simulink model "C_PTES_sim_v2"  (R2025a)
settings: Solver=ode23tb  StartTime=0.0  StopTime=600
PreLoadFcn:
  | Load_Maps
InitFcn:
  | A_init_compressor
StopFcn:
  | % AB_plotHX
  | % AB_plotmap
model workspace (MAT data in the model file):
  Step_time = 1000
  step_time = 200
values from neighbouring files (symbols this model uses):
  DeltaW = 0    [A_init_compressor.m]    (also in B_init_compressor.m = input('Power change: '))
  Ki_tau = 23.1297    [A_init_compressor.m]    (also in B_init_compressor.m = 0.1)
  Kp_tau = 289.6844    [A_init_compressor.m]    (also in B_init_compressor.m = 1)
  omega_step = 376    [A_init_compressor.m]
  stepping_time = 100000    [A_init_compressor.m]    (also in B_init_compressor.m = input('Step time:'))
  tchange = 100000    [A_init_compressor.m]
undefined symbols (not defined in the file or in its folder): z_Qlty_CO2
libraries: simulink_extras x17, slpidlib x9
(part 1 of 3)
settings Model: Creator=mmercang  LastModifiedBy=alpalbay
settings SolverCC: ConsecutiveZCsStepRelTol=auto  ZeroCrossAlgorithm=Adaptive  MinimalZcImpactIntegration=on
settings DataIOCC: FinalStateName=xfinal  InitialState=steady_state  LoadInitialState=on  SaveFinalState=on  SaveFormat=StructureWithTime  SaveState=on  Refine=2
settings DebuggingCC: ReadBeforeWriteMsg=DisableAll  WriteAfterWriteMsg=DisableAll  WriteAfterReadMsg=DisableAll  AlgebraicLoopMsg=none  IgnoredZcDiagnostic=none  MultiTaskDSMMsg=none
settings ModelReferenceCC: UpdateModelReferenceTargets=IfOutOfDate
settings SFSimCC: SFSimEcho=off
settings RTWCC: GPUComputeCapability=3.5
settings SimscapeCC: SimscapeLogDecimation=1  SimscapeLogDataHistory=5000

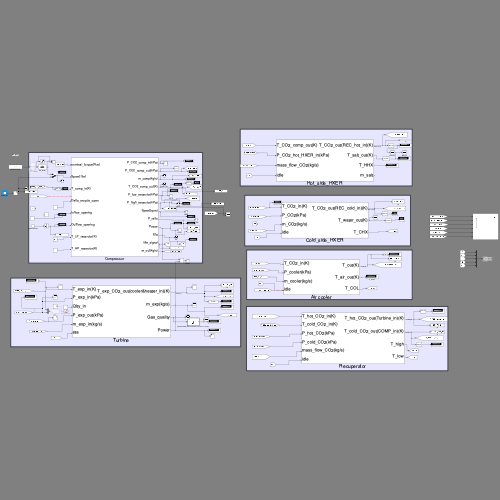
[thumbnail: Simulink's stored preview of the top-level diagram]
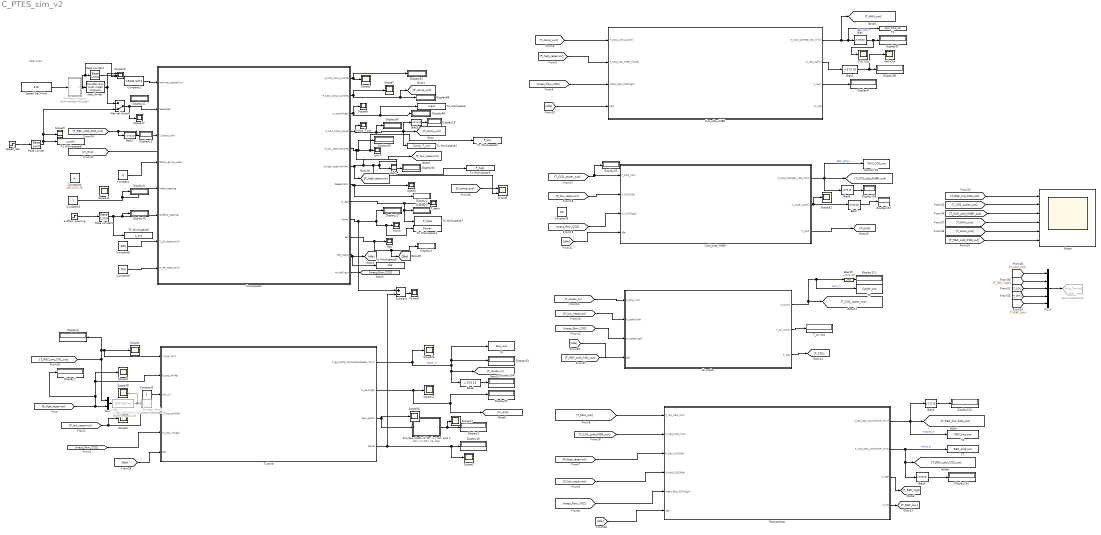
== system C_PTES_sim_v2 ==
  note: 368.2243
  Air cooler : Subsystem
  Bias{,1..8,15} (10 alike) : Bias  Bias=-273.15  SaturateOnIntegerOverflow=off
  CO2 Out : Scope
      settings: ActiveDisplayYMinimum=419.41887849810757  ActiveDisplayYMaximum=425.62012461132127  DataLoggingVariableName=ScopeData57
  Cold_side_HXER : Subsystem
  Comp T out : Scope
      settings: ActiveDisplayYMinimum=932.8388554275466  ActiveDisplayYMaximum=966.06264783948268  DataLoggingVariableName=ScopeData42
  Compressor : Subsystem
  Constant : Constant  Value=0
  Constant1 : Constant  Value=19102.6473
  Constant2 : Constant
  Constant3 : Constant
  Constant4 : Constant  Value=420+273.15
  Constant5 : Constant  Value=50
  Constant8 : Constant  Value=690
  Constant9 : Constant  Value=700
  Display{1..4,6..13,16,19..20,87..94,97..98,101..102,104,107..108,113} (31 alike) : Display
      Display12 settings: Format=bank
  Dryness check : MATLAB Function  Commented=on  TreatAsAtomicUnit=on
  "Dryness check (0 for \"x<=0\" and 1 for \"x>=1\" i.e. dry)" : MATLAB Function  TreatAsAtomicUnit=on
  Eta : Scope
      settings: ActiveDisplayYMinimum=0.8  ActiveDisplayYMaximum=1  DataLoggingVariableName=ScopeData44
  Goto17 : Goto  Commented=on  GotoTag=Avg_Temps
  High P : Scope
      settings: ActiveDisplayYMinimum=19499.01131682  ActiveDisplayYMaximum=19499.01131709  DataLoggingVariableName=ScopeData45
  Hot_side_HXER : Subsystem
  Low P : Scope
      settings: ActiveDisplayYMinimum=1661.4124691306079  ActiveDisplayYMaximum=8047.2877774228209  DataLoggingVariableName=ScopeData46
  Manual Switch : ManualSwitch  CurrentSetting=0
  Mux : Mux  Inputs=2
  Mux1 : Mux  Inputs=5
  P_ratio : Scope
      settings: ActiveDisplayYMinimum=2.5704663897454543  ActiveDisplayYMaximum=2.6288728670169967  DataLoggingVariableName=ScopeData47
  Power : Scope
      settings: ActiveDisplayYMinimum=9622.94144984568  ActiveDisplayYMaximum=9622.9443761527218  DataLoggingVariableName=ScopeData48
  Power1 : Scope
      settings: ActiveDisplayYMinimum=-764.83256469030607  ActiveDisplayYMaximum=6887.6317450574907  DataLoggingVariableName=ScopeData84
  Qlty : MATLABFcn  Commented=on  MATLABFcn=z_Qlty_CO2(u(1),u(2))
  Rate Limiter : RateLimiter
  Rate Limiter1 : RateLimiter  RisingSlewLimit=4  FallingSlewLimit=-4  InitialCondition=376  LinearizeAsGain=off
  Rate Limiter2 : RateLimiter  FallingSlewLimit=-0.01
  Recuperator : Subsystem
  Salt Out : Scope
      settings: ActiveDisplayYMinimum=549.32679199371159  ActiveDisplayYMaximum=549.32679200120469  DataLoggingVariableName=ScopeData58
  Scope : Scope  NumInputPorts=6
      settings: ActiveDisplayYMinimum=408.50778721774293  ActiveDisplayYMaximum=410.82110455322322
  Scope{1..5,7..9,11,17,22..23,26..28,51} (16 alike) : Scope
      Scope1 settings: ActiveDisplayYMinimum=354.53484488928774  ActiveDisplayYMaximum=416.54773222280147
      Scope11 settings: ActiveDisplayYMinimum=0.043750000000000011  ActiveDisplayYMaximum=1.10625  DataLoggingVariableName=ScopeData15
      Scope17 settings: ActiveDisplayYMinimum=346.2691444179722  ActiveDisplayYMaximum=643.57770023825037  DataLoggingVariableName=ScopeData49
      Scope2 settings: ActiveDisplayYMinimum=3609.0647035085312  ActiveDisplayYMaximum=3633.4611371786241
      Scope22 settings: ActiveDisplayYMinimum=53.375645074893505  ActiveDisplayYMaximum=53.375742212262359  DataLoggingVariableName=ScopeData5
      Scope23 settings: ActiveDisplayYMinimum=249.61773578013822  ActiveDisplayYMaximum=330.2583181291364  DataLoggingVariableName=ScopeData6
      Scope26 settings: ActiveDisplayYMinimum=-1  ActiveDisplayYMaximum=1
      Scope27 settings: ActiveDisplayYMinimum=-1  ActiveDisplayYMaximum=1  DataLoggingVariableName=ScopeData2
      Scope28 settings: ActiveDisplayYMinimum=-1  ActiveDisplayYMaximum=1  DataLoggingVariableName=ScopeData3
      Scope3 settings: ActiveDisplayYMinimum=6922.0923934778948  ActiveDisplayYMaximum=12119.561569977996  DataLoggingVariableName=ScopeData50
      Scope4 settings: ActiveDisplayYMinimum=19499.011316899083  ActiveDisplayYMaximum=19499.011316899174  DataLoggingVariableName=ScopeData5
      Scope5 settings: ActiveDisplayYMinimum=7403.99999999722  ActiveDisplayYMaximum=7404.0000000235223  DataLoggingVariableName=ScopeData6
      Scope51 settings: ActiveDisplayYMinimum=252.25553854956786  ActiveDisplayYMaximum=331.783751710615  DataLoggingVariableName=ScopeData2
      Scope7 settings: ActiveDisplayYMinimum=-9616.8305551512967  ActiveDisplayYMaximum=198282.22438144876  DataLoggingVariableName=ScopeData52
      Scope8 settings: ActiveDisplayYMinimum=53.375694282294106  ActiveDisplayYMaximum=53.37575539188817  DataLoggingVariableName=ScopeData53
      Scope9 settings: ActiveDisplayYMinimum=276  ActiveDisplayYMaximum=476  DataLoggingVariableName=ScopeData85
  Scope10 : Scope  NumInputPorts=3
      settings: ActiveDisplayYMinimum=375.99999999999989  ActiveDisplayYMaximum=376.00000000000011  DataLoggingVariableName=ScopeData10
  Scope6 : Scope  NumInputPorts=2
      settings: ActiveDisplayYMinimum=724.91071659726686  ActiveDisplayYMaximum=20997.430200370087  DataLoggingVariableName=ScopeData55
  Shutdown Signal : Subsystem  Commented=through
  Speed : Scope
      settings: ActiveDisplayYMinimum=375.99998147375209  ActiveDisplayYMaximum=376.00015418573196  DataLoggingVariableName=ScopeData54
  Speed Set Point : Constant  Value=376
  Speed_Set : Step  Time=stepping_time  Before=376  After=omega_step  SampleTime=0
  Subtract : Sum  Inputs=+-
  T1 : ToWorkspace  VariableName=HHX_CO2_out  SampleTime=-1
      settings: Save2DSignal=2-D array (concatenate along first dimension)
  T3 : ToWorkspace  VariableName=REC_hot_out  SampleTime=-1
      settings: Save2DSignal=2-D array (concatenate along first dimension)
  T4 : ToWorkspace  VariableName=Exp_out  SampleTime=-1
      settings: Save2DSignal=2-D array (concatenate along first dimension)
  T5 : ToWorkspace  VariableName=Cooler_out  SampleTime=-1
      settings: Save2DSignal=2-D array (concatenate along first dimension)
  T6 : ToWorkspace  VariableName=CHX_CO2_out  SampleTime=-1
      settings: Save2DSignal=2-D array (concatenate along first dimension)
  T7 : ToWorkspace  VariableName=REC_cold_out  SampleTime=-1
      settings: Save2DSignal=2-D array (concatenate along first dimension)
  T_air Out : Display
  To Workspace : ToWorkspace  VariableName=mass  SampleTime=-1
      settings: Save2DSignal=2-D array (concatenate along first dimension)
  To Workspace1 : ToWorkspace  VariableName=Power  SampleTime=-1
      settings: Save2DSignal=2-D array (concatenate along first dimension)
  To Workspace2 : ToWorkspace  VariableName=Comp_T_out  SampleTime=-1
      settings: Save2DSignal=2-D array (concatenate along first dimension)
  To Workspace3 : ToWorkspace  VariableName=P_high  SampleTime=-1
      settings: Save2DSignal=2-D array (concatenate along first dimension)
  To Workspace4 : ToWorkspace  VariableName=P_low  SampleTime=-1
      settings: Save2DSignal=2-D array (concatenate along first dimension)
  To Workspace5 : ToWorkspace  VariableName=z_out  SampleTime=-1
      settings: Save2DSignal=2-D array (concatenate along first dimension)
  To Workspace6 : ToWorkspace  VariableName=idle  SampleTime=-1
      settings: Save2DSignal=2-D array (concatenate along first dimension)
  To Workspace7 : ToWorkspace  VariableName=P_ratio  SampleTime=-1
      settings: Save2DSignal=2-D array (concatenate along first dimension)
  To Workspace8 : ToWorkspace  VariableName=z_out1  SampleTime=-1
      settings: Save2DSignal=2-D array (concatenate along first dimension)
  Turbine : Subsystem
  outflow opening : Step  Time=10000  Before=1  SampleTime=0
  rate_limiter : simulink_extras/Additional Linear/Transfer Fcn (with initial outputs)  N=[1]  D="[30  1]"  Y0=376  U0=0
  wires:
  [mass_flow_CO2] -> Turbine/5(m_exp_in(kg/s))
  [T_HHX_out] -> Recuperator/1(T_hot_CO2_in(K))
  [P_high_reservoir] -> Recuperator/3(P_hot_CO2(kPa))
  [P_low_reservoir] -> Recuperator/4(P_cold_CO2(kPa))
  [mass_flow_CO2] -> Recuperator/5(mass_flow_CO2(kg/s))
  Bias4/1 -> Display101/1
  Bias5/1 -> Display102/1
  [mass_flow_CO2] -> Air cooler/3(m_cooler(kg/s))
  [P_low_reservoir] -> Air cooler/2(P_cooler(kPa))
  Bias15/1 -> Display113/1
  Air cooler/1(T_out(K)) -> Bias15/1, T5/1, [T_CO2_cooler_out]  "CHX_in"
  Bias6/1 -> Display104/1
  [T_CO2_cooler_out] -> Display20/1, Cold_side_HXER/1(T_CO2_in(K))
  [P_low_reservoir] -> Cold_side_HXER/2(P_CO2(kPa))
  Cold_side_HXER/1(T_CO2_out(REC_cold_in)(K)) -> T6/1, [T_CO2_cold_HXER_out], Bias8/1  "REC_cold_in"
  Cold_side_HXER/2(T_water_out(K)) -> Scope51/1, Bias7/1
  Bias7/1 -> Display107/1
  Bias8/1 -> Display108/1
  [T_CO2_cold_HXER_out] -> Recuperator/2(T_cold_CO2_in(K))
  Recuperator/1(T_hot_CO2_out(Turbine_in)(K)) -> Bias4/1, T3/1, [T_REC_hot_CO2_out]  "Turbine_in"
  Recuperator/2(T_cold_CO2_out(COMP_in)(K)) -> Bias5/1, [T_REC_cold_CO2_out], T7/1  "Comp_in"
  Turbine/3(Gas_quality) -> "Dryness check (0 for \"x<=0\" and 1 for \"x>=1\" i.e. dry)"/1(u), Scope26/1
  Qlty/1 -> Dryness check/1(u), Scope28/1
  Mux/1 -> Qlty/1
  [P_high_reservoir] -> Display7/1, Scope4/1, Turbine/2(P_exp_in(kPa)), Mux/2
  Turbine/1(T_exp_CO2_out(cooler&heater_in)(K)) -> Bias6/1, [T_cooler_in], T4/1, Display91/1, Scope23/1  "Cooler_in"
  Turbine/2(m_exp(kg/s)) -> Display92/1, [m_exp], Scope22/1
  [T_REC_hot_CO2_out] -> Display6/1, Turbine/1(T_exp_in(K)), Scope1/1, Mux/1
  [P_low_reservoir] -> Turbine/4(P_exp_out(kPa)), Scope5/1
  [T_cooler_in] -> Air cooler/1(T_CO2_in(K))
  [T_REC_hot_CO2_out] -> Scope/1
  [T_HHX_out] -> Scope/4
  [T_CO2_cooler_out] -> Scope/2
  [T_CO2_cold_HXER_out] -> Scope/3
  [T_REC_cold_CO2_out] -> Scope/6
  [T_comp_out] -> Scope/5
  "Dryness check (0 for \"x<=0\" and 1 for \"x>=1\" i.e. dry)"/1(y) -> Scope27/1, Display2/1
  Turbine/4(Power) -> Subtract/2, Scope2/1, Display16/1
  Air cooler/2(T_air_out(K)) -> T_air Out/1
  [Eta] -> Turbine/6(eta)
  Recuperator/3(T_high) -> [T_REC_high]
  Recuperator/4(T_low) -> [T_REC_low]
  Air cooler/3(T_COL) -> [T_COL]
  [T_HHX_out] -> Mux1/1
  [T_REC_high] -> Mux1/2
  [T_COL] -> Mux1/3
  [T_CHX] -> Mux1/4
  [T_REC_low] -> Mux1/5
  Mux1/1 -> Goto17/1
  Compressor/10(Eta) -> Eta/1, [Eta], Display4/1
  [m_exp] -> ?
  Bias2/1 -> Display13/1
  Bias1/1 -> Display19/1
  Manual Switch/1 -> Scope17/1, Compressor/2(Speed Set)
  Constant3/1 -> Display9/1, Compressor/5(Inflow_opening)
  Compressor/5(P_low_reservior(kPa)) -> [P_low_reservoir], To Workspace4/1, Low P/1, Display93/1
  Compressor/12(m_out(kg/s)) -> [mass_flow_CO2]
  Compressor/7(Speed(rpm)) -> Display1/1, Speed/1
  Shutdown Signal/1(Out1) -> Scope10/3, Rate Limiter1/1, rate_limiter/1
  Compressor/8(P_ratio) -> P_ratio/1, To Workspace7/1, Display3/1
  Constant8/1 -> Compressor/7(T_LP_reservior(K))
  Compressor/1(P_CO2_comp_in(kPa)) -> Scope3/1, Display87/1
  Compressor/2(P_CO2_comp_out(kPa)) -> [P_comp_out], Display88/1, Scope7/1
  Compressor/11(idle_signal) -> To Workspace6/1, [idle]
  [T_REC_cold_CO2_out] -> Bias2/1, Compressor/3(T_comp_in(K))
  Constant/1 -> Compressor/4(Delta_recycle_open)
  Speed Set Point/1 -> Shutdown Signal/1(In1)
  outflow opening/1 -> Rate Limiter2/1
  Constant1/1 -> Compressor/1(nominal_torque(N.m))
  Compressor/9(Power) -> To Workspace1/1, Power/1, Display12/1, Subtract/1
  Compressor/3(m_comp(kg/s)) -> To Workspace/1, Display89/1, Scope8/1
  Compressor/6(P_high_reservior(kPa)) -> [P_high_reservoir], To Workspace3/1, Scope6/2, High P/1, Display94/1
  Compressor/4(T_CO2_comp_out(K)) -> [T_comp_out], Bias1/1, To Workspace2/1, Display90/1, Comp T out/1
  Constant9/1 -> Compressor/8(T_HP_reservior(K))
  [P_comp_out] -> Scope6/1
  [idle] -> Hot_side_HXER/4(idle)
  Hot_side_HXER/3(T_HHX) -> Display8/1
  Bias3/1 -> Salt Out/1, Display98/1
  [P_high_reservoir] -> Hot_side_HXER/2(P_CO2_hot_HXER_in(kPa))
  [T_comp_out] -> Hot_side_HXER/1(T_CO2_comp_out(K))
  Bias/1 -> CO2 Out/1, Display97/1
  [mass_flow_CO2] -> Hot_side_HXER/3(mass_flow_CO2(kg/s))
  Hot_side_HXER/2(T_salt_out(K)) -> Bias3/1
  Hot_side_HXER/1(T_CO2_out(REC_hot_in)(K)) -> [T_HHX_out], T1/1, Bias/1  "REC_Hot_in"
  [idle] -> Cold_side_HXER/4(idle)
  Constant2/1 -> Turbine/3(Qlty_in)
  [mass_flow_CO2] -> Cold_side_HXER/3(m_CO2(kg/s))
  Subtract/1 -> Power1/1
  Cold_side_HXER/3(T_CHX) -> [T_CHX]
  Speed_Set/1 -> Rate Limiter/1
  rate_limiter/1 -> Manual Switch/1, Scope10/1
  Rate Limiter1/1 -> Scope10/2
  [idle] -> Recuperator/6(idle)
  Rate Limiter2/1 -> To Workspace5/1, Compressor/6(Outflow_opening), Display10/1
  [T_REC_cold_CO2_out] -> ?
  [idle] -> Air cooler/4(idle)
  Rate Limiter/1 -> Scope9/1, Manual Switch/2, To Workspace8/1

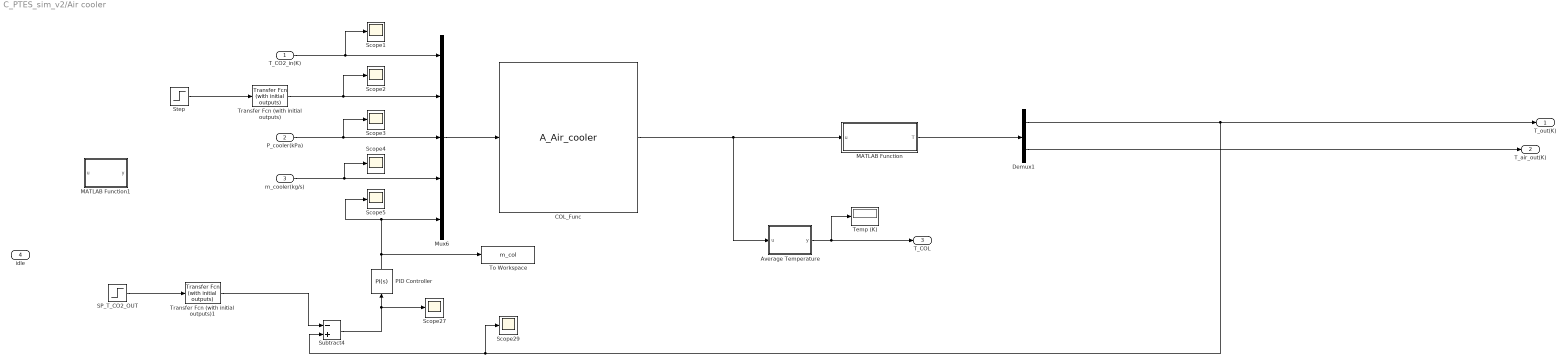
== system C_PTES_sim_v2/Air cooler ==
  T_CO2_in(K) : Inport
  P_cooler(kPa) : Inport  Port=2
  m_cooler(kg/s) : Inport  Port=3
  idle : Inport  Port=4
  Average Temperature : MATLAB Function  TreatAsAtomicUnit=on
  COL_Func : S-Function  InitFcn=A_init_HXERs  FunctionName=A_Air_cooler  Parameters=Param  SFunctionDeploymentMode=off  EnableBusSupport=off
  Demux1 : Demux  Outputs=2
  MATLAB Function : MATLAB Function  TreatAsAtomicUnit=on
  MATLAB Function1 : MATLAB Function  TreatAsAtomicUnit=on
  Mux6 : Mux  Inputs=5
  PID Controller : slpidlib/PID Controller  Controller=PI  Form=Parallel  TimeDomain=Continuous-time  UseExternalTs=off  SampleTime=-1  IntegratorMethod=Forward Euler  FilterMethod=Forward Euler  ControllerParametersSource=internal  P=5  I=0.4  UseKiTs=off  D=0  UseExternalDerivativeSource=off  N=1  UseFilter=on  TunerSelectOption=Transfer Function Based (PID Tuner App)  InitialConditionSource=internal  InitialConditionForIntegrator=0  InitialConditionForFilter=0  DifferentiatorICPrevScaledInput=0  ExternalReset=none  TrackingMode=off  Kt=1  LimitOutput=on  SatLimitsSource=internal  UpperSaturationLimit=10000000  LowerSaturationLimit=0  LinearizeAsGain=off  AntiWindupMode=back-calculation  Kb=10  LimitIntegrator=off  UpperIntegratorSaturationLimit=inf  LowerIntegratorSaturationLimit=-inf  POutMin=[]  POutMax=[]  IOutMin=[]  IOutMax=[]  DOutMin=[]  DOutMax=[]  NOutMin=[]  NOutMax=[]  SumOutMin=[]  SumOutMax=[]  SaturationOutMin=[]  SaturationOutMax=[]  PParamMin=[]  PParamMax=[]  IParamMin=[]  IParamMax=[]  DParamMin=[]  DParamMax=[]  NParamMin=[]  NParamMax=[]  KbParamMin=[]  KbParamMax=[]  KtParamMin=[]  KtParamMax=[]  KbOutMin=[]  KbOutMax=[]  KtOutMin=[]  KtOutMax=[]  IntegratorOutMin=[]  IntegratorOutMax=[]  FilterOutMin=[]  FilterOutMax=[]  SumI1OutMin=[]  SumI1OutMax=[]  SumI2OutMin=[]  SumI2OutMax=[]  SumI3OutMin=[]  SumI3OutMax=[]  SumI4OutMin=[]  SumI4OutMax=[]  SumDOutMin=[]  SumDOutMax=[]  DifferentiatorOutMin=[]  DifferentiatorOutMax=[]  FilterDiffOutCoefMin=[]  FilterDiffOutCoefMax=[]  ReciprocalOutMin=[]  ReciprocalOutMax=[]  SumDenOutMin=[]  SumDenOutMax=[]  SumNumOutMin=[]  SumNumOutMax=[]  DivideOutMin=[]  DivideOutMax=[]  UdiffTsProdOutMin=[]  UdiffTsProdOutMax=[]  NTsProdOutMin=[]  NTsProdOutMax=[]  UintegralTsProdOutMin=[]  UintegralTsProdOutMax=[]  UngainTsProdOutMin=[]  UngainTsProdOutMax=[]  ClampingZeroOutDataTypeStr=Inherit: Inherit via back propagation  ClampingZeroOutMin=[]  ClampingZeroOutMax=[]  FilterDenConstantOutDataTypeStr=Inherit: Inherit via back propagation  FilterDenConstantOutMin=[]  FilterDenConstantOutMax=[]  PCopyOutDataTypeStr=Inherit: Inherit via back propagation  PCopyOutMin=[]  PCopyOutMax=[]  NCopyOutDataTypeStr=Inherit: Inherit via back propagation  NCopyOutMin=[]  NCopyOutMax=[]  IntegratorContinuousStateAttributes=''  IntegratorStateMustResolveToSignalObject=off  IntegratorRTWStateStorageClass=Auto  FilterContinuousStateAttributes=''  FilterStateMustResolveToSignalObject=off  FilterRTWStateStorageClass=Auto  ParallelPVariant=InternalParameters  IdealPVariant=Disabled  IVariant=InternalParameters  DVariant=Disabled  IntegratorVariant=Continuous  SatVariant=Enabled  AWVariant=BackCalculation  PCopyVariant=Disabled  TRVariant=Disabled  FdbkBlocksVariant=Forward  IdealPFdbkVariant=Disabled  SatFdbkVariant=Disabled  DerivativeFilterVariant=Disabled  NVariant=Disabled  NCopyVariant=Disabled_SignalSpec  FilterICVariant=Disabled  IntegratorICVariant=InternalICs  ExternalResetVariant=Disabled  TRSumVariant=Passthrough  SumFdbkVariant=Disabled  SumVariant=Sum_PI  TsampFilterVariant=InternalTs  TsampNgainVariant=Passthrough  TsampIntegralVariant=Disabled_SignalSpec  ExternalSaturationOutDataTypeStr=Inherit: Same as second input  DerivativeSourceVariant=Disabled  PreIntVariant=InternalPreInt
  SP_T_CO2_OUT : Step  Time=tchange  Before=320  After=262  SampleTime=0
  Scope{1..5,27,29} (7 alike) : Scope
      Scope1 settings: ActiveDisplayYMinimum=250.86972804134678  ActiveDisplayYMaximum=327.89638764837019
      Scope2 settings: ActiveDisplayYMinimum=193.15  ActiveDisplayYMaximum=393.15  DataLoggingVariableName=ScopeData2
      Scope27 settings: ActiveDisplayYMinimum=-37.044023747465346  ActiveDisplayYMaximum=4.1159882470852116  DataLoggingVariableName=ScopeData90
      Scope29 settings: ActiveDisplayYMinimum=250.50677583981667  ActiveDisplayYMaximum=327.76502730783477  DataLoggingVariableName=ScopeData92
      Scope3 settings: ActiveDisplayYMinimum=7547.995411  ActiveDisplayYMaximum=7547.995423  DataLoggingVariableName=ScopeData3
      Scope4 settings: ActiveDisplayYMinimum=47.13636  ActiveDisplayYMaximum=47.59275  DataLoggingVariableName=ScopeData4
      Scope5 settings: ActiveDisplayYMinimum=-70.947895404944461  ActiveDisplayYMaximum=638.53105864450026
  Step : Step  Time=tchange  Before=20+273.15  After=-30+273.15  SampleTime=0
  Subtract4 : Sum  Inputs=-+
  Temp (K) : Display
  To Workspace : ToWorkspace  VariableName=m_col  SaveFormat=Timeseries  SampleTime=-1
  Transfer Fcn (with initial outputs) : simulink_extras/Additional Linear/Transfer Fcn (with initial outputs)  N=[1]  D="[5  1]"  Y0=20+273.15  U0=0
  Transfer Fcn (with initial outputs)1 : simulink_extras/Additional Linear/Transfer Fcn (with initial outputs)  N=[1]  D="[5  1]"  Y0=320  U0=0
  T_out(K) : Outport
  T_air_out(K) : Outport  Port=2
  T_COL : Outport  Port=3
  wires:
  m_cooler(kg/s)/1 -> Mux6/4, Scope4/1
  P_cooler(kPa)/1 -> Scope3/1, Mux6/3
  Mux6/1 -> COL_Func/1
  Step/1 -> Transfer Fcn (with initial outputs)/1
  T_CO2_in(K)/1 -> Scope1/1, Mux6/1
  PID Controller/1 -> Scope5/1, Mux6/5, To Workspace/1
  Demux1/1 -> Subtract4/2, Scope29/1, T_out(K)/1
  Demux1/2 -> T_air_out(K)/1
  MATLAB Function/1(T) -> Demux1/1
  Average Temperature/1(y) -> Temp (K)/1, T_COL/1
  COL_Func/1 -> Average Temperature/1(u), MATLAB Function/1(u)
  Subtract4/1 -> Scope27/1, PID Controller/1
  SP_T_CO2_OUT/1 -> Transfer Fcn (with initial outputs)1/1
  Transfer Fcn (with initial outputs)/1 -> Scope2/1, Mux6/2
  Transfer Fcn (with initial outputs)1/1 -> Subtract4/1

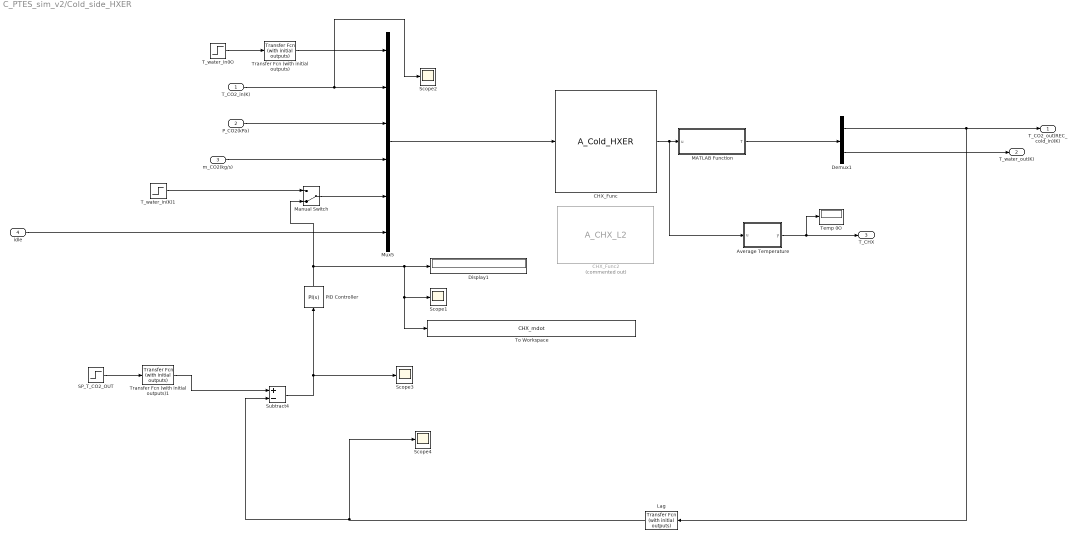
== system C_PTES_sim_v2/Cold_side_HXER ==
  T_CO2_in(K) : Inport
  P_CO2(kPa) : Inport  Port=2
  m_CO2(kg/s) : Inport  Port=3
  idle : Inport  Port=4
  Average Temperature : MATLAB Function  TreatAsAtomicUnit=on
  CHX_Func : S-Function  FunctionName=A_Cold_HXER  Parameters=Param  SFunctionDeploymentMode=off  EnableBusSupport=off
  CHX_Func2 : M-S-Function  Commented=on  FunctionName=A_CHX_L2  Parameters=Param
  Demux1 : Demux  Outputs=2
  Display1 : Display
      settings: Format=long_e
  Lag : simulink_extras/Additional Linear/Transfer Fcn (with initial outputs)  N=[1]  D="[2  1]"  Y0=90+273.15  U0=0
  MATLAB Function : MATLAB Function  TreatAsAtomicUnit=on
  Manual Switch : ManualSwitch  CurrentSetting=0
  Mux5 : Mux  Inputs=6
  PID Controller : slpidlib/PID Controller  Controller=PI  Form=Parallel  TimeDomain=Continuous-time  UseExternalTs=off  SampleTime=-1  IntegratorMethod=Forward Euler  FilterMethod=Forward Euler  ControllerParametersSource=internal  P=1  I=0.5  UseKiTs=off  D=0  UseExternalDerivativeSource=off  N=1  UseFilter=on  TunerSelectOption=Transfer Function Based (PID Tuner App)  InitialConditionSource=internal  InitialConditionForIntegrator=0  InitialConditionForFilter=0  DifferentiatorICPrevScaledInput=0  ExternalReset=none  TrackingMode=off  Kt=1  LimitOutput=on  SatLimitsSource=internal  UpperSaturationLimit=1000  LowerSaturationLimit=0  LinearizeAsGain=off  AntiWindupMode=back-calculation  Kb=10  LimitIntegrator=off  UpperIntegratorSaturationLimit=inf  LowerIntegratorSaturationLimit=-inf  POutMin=[]  POutMax=[]  IOutMin=[]  IOutMax=[]  DOutMin=[]  DOutMax=[]  NOutMin=[]  NOutMax=[]  SumOutMin=[]  SumOutMax=[]  SaturationOutMin=[]  SaturationOutMax=[]  PParamMin=[]  PParamMax=[]  IParamMin=[]  IParamMax=[]  DParamMin=[]  DParamMax=[]  NParamMin=[]  NParamMax=[]  KbParamMin=[]  KbParamMax=[]  KtParamMin=[]  KtParamMax=[]  KbOutMin=[]  KbOutMax=[]  KtOutMin=[]  KtOutMax=[]  IntegratorOutMin=[]  IntegratorOutMax=[]  FilterOutMin=[]  FilterOutMax=[]  SumI1OutMin=[]  SumI1OutMax=[]  SumI2OutMin=[]  SumI2OutMax=[]  SumI3OutMin=[]  SumI3OutMax=[]  SumI4OutMin=[]  SumI4OutMax=[]  SumDOutMin=[]  SumDOutMax=[]  DifferentiatorOutMin=[]  DifferentiatorOutMax=[]  FilterDiffOutCoefMin=[]  FilterDiffOutCoefMax=[]  ReciprocalOutMin=[]  ReciprocalOutMax=[]  SumDenOutMin=[]  SumDenOutMax=[]  SumNumOutMin=[]  SumNumOutMax=[]  DivideOutMin=[]  DivideOutMax=[]  UdiffTsProdOutMin=[]  UdiffTsProdOutMax=[]  NTsProdOutMin=[]  NTsProdOutMax=[]  UintegralTsProdOutMin=[]  UintegralTsProdOutMax=[]  UngainTsProdOutMin=[]  UngainTsProdOutMax=[]  ClampingZeroOutDataTypeStr=Inherit: Inherit via back propagation  ClampingZeroOutMin=[]  ClampingZeroOutMax=[]  FilterDenConstantOutDataTypeStr=Inherit: Inherit via back propagation  FilterDenConstantOutMin=[]  FilterDenConstantOutMax=[]  PCopyOutDataTypeStr=Inherit: Inherit via back propagation  PCopyOutMin=[]  PCopyOutMax=[]  NCopyOutDataTypeStr=Inherit: Inherit via back propagation  NCopyOutMin=[]  NCopyOutMax=[]  IntegratorContinuousStateAttributes=''  IntegratorStateMustResolveToSignalObject=off  IntegratorRTWStateStorageClass=Auto  FilterContinuousStateAttributes=''  FilterStateMustResolveToSignalObject=off  FilterRTWStateStorageClass=Auto  ParallelPVariant=InternalParameters  IdealPVariant=Disabled  IVariant=InternalParameters  DVariant=Disabled  IntegratorVariant=Continuous  SatVariant=Enabled  AWVariant=BackCalculation  PCopyVariant=Disabled  TRVariant=Disabled  FdbkBlocksVariant=Forward  IdealPFdbkVariant=Disabled  SatFdbkVariant=Disabled  DerivativeFilterVariant=Disabled  NVariant=Disabled  NCopyVariant=Disabled_SignalSpec  FilterICVariant=Disabled  IntegratorICVariant=InternalICs  ExternalResetVariant=Disabled  TRSumVariant=Passthrough  SumFdbkVariant=Disabled  SumVariant=Sum_PI  TsampFilterVariant=InternalTs  TsampNgainVariant=Passthrough  TsampIntegralVariant=Disabled_SignalSpec  ExternalSaturationOutDataTypeStr=Inherit: Same as second input  DerivativeSourceVariant=Disabled  PreIntVariant=InternalPreInt
  SP_T_CO2_OUT : Step  Time=tchange  Before=361.15  After=20+273.15  SampleTime=0
  Scope{1..4} (4 alike) : Scope
      Scope1 settings: ActiveDisplayYMinimum=17.380675439645675  ActiveDisplayYMaximum=64.3264765007091
      Scope2 settings: ActiveDisplayYMinimum=301.50681711475363  ActiveDisplayYMaximum=322.05478370683869  DataLoggingVariableName=ScopeData8
      Scope3 settings: ActiveDisplayYMinimum=-0.25130005631149993  ActiveDisplayYMaximum=2.2617131375430475  DataLoggingVariableName=ScopeData3
      Scope4 settings: ActiveDisplayYMinimum=-1  ActiveDisplayYMaximum=1  DataLoggingVariableName=ScopeData4
  Subtract4 : Sum  Inputs=+-
  T_water_in(K) : Step  Time=tchange  Before=90+273.15  After=21+273.15  SampleTime=0
  T_water_in(K)1 : Step  Time=1e9  After=0  SampleTime=0
  Temp (K) : Display
  To Workspace : ToWorkspace  VariableName=CHX_mdot  SampleTime=-1
  Transfer Fcn (with initial outputs) : simulink_extras/Additional Linear/Transfer Fcn (with initial outputs)  N=[1]  D="[5  1]"  Y0=90+273.15  U0=0
  Transfer Fcn (with initial outputs)1 : simulink_extras/Additional Linear/Transfer Fcn (with initial outputs)  N=[1]  D="[5  1]"  Y0=88 + 273.15  U0=0
  T_CO2_out(REC_cold_in)(K) : Outport
  T_water_out(K) : Outport  Port=2
  T_CHX : Outport  Port=3
  wires:
  P_CO2(kPa)/1 -> Mux5/3
  m_CO2(kg/s)/1 -> Mux5/4
  T_CO2_in(K)/1 -> Scope2/1, Mux5/2
  T_water_in(K)/1 -> Transfer Fcn (with initial outputs)/1
  PID Controller/1 -> Display1/1, Scope1/1, To Workspace/1, Manual Switch/2
  Subtract4/1 -> Scope3/1, PID Controller/1
  MATLAB Function/1(T) -> Demux1/1
  Demux1/2 -> T_water_out(K)/1
  Demux1/1 -> Lag/1, T_CO2_out(REC_cold_in)(K)/1
  Mux5/1 -> CHX_Func/1
  Average Temperature/1(y) -> T_CHX/1, Temp (K)/1
  CHX_Func/1 -> MATLAB Function/1(u), Average Temperature/1(u)
  idle/1 -> Mux5/6
  SP_T_CO2_OUT/1 -> Transfer Fcn (with initial outputs)1/1
  T_water_in(K)1/1 -> Manual Switch/1
  Manual Switch/1 -> Mux5/5
  Lag/1 -> Scope4/1, Subtract4/2
  Transfer Fcn (with initial outputs)/1 -> Mux5/1
  Transfer Fcn (with initial outputs)1/1 -> Subtract4/1
